simulink model "Ford_T3T6_ArchCnctnDigrm"  (R2016b)
settings: Solver=FixedStepDiscrete  StartTime=0.0  StopTime=10.0  RelTol=1e-3  EnableMultiTasking=on
libraries: canmsglib x15
(part 6 of 15)

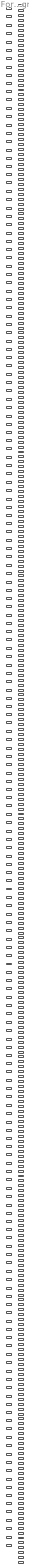
== system Ford_T3T6_ArchCnctnDigrm/Motor Control Manager/AR300FORDA_MotCtrlMgr ==
  AdcDiagcEndPtrOutp : Inport
  AdcDiagcStrtPtrOutp : Inport  Port=2
  BrdgVltg : Inport  Port=3
  CtrlrTFild : Inport  Port=4
  CurrMeasCorrlnSts : Inport  Port=5
  CurrMeasLoaMtgtnEna : Inport  Port=6
  DiagcStsIvtr1Inactv : Inport  Port=7
  DiagcStsIvtr2Inactv : Inport  Port=8
  DualEcuMotCtrlMtgtnEna : Inport  Port=9
  EcuTFild : Inport  Port=10
  HwTq4Raw : Inport  Port=11
  HwTq5Raw : Inport  Port=12
  IvtrFetFltPha : Inport  Port=13
  IvtrFetFltTyp : Inport  Port=14
  IvtrLoaMtgtnEna : Inport  Port=15
  LoopCntr2MilliSec : Inport  Port=16
  MfgEnaSt : Inport  Port=17
  MotAg0ABIFaild : Inport  Port=18
  MotAg0Offs : Inport  Port=19
  MotAg0QepFaild : Inport  Port=20
  MotAg1ABIFaild : Inport  Port=21
  MotAg1Offs : Inport  Port=22
  MotAg1QepFaild : Inport  Port=23
  MotAg2Cos : Inport  Port=24
  MotAg2CosAdcFaild : Inport  Port=25
  MotAg2Sin : Inport  Port=26
  MotAg2SinAdcFaild : Inport  Port=27
  MotAg5CosAdcFaild : Inport  Port=28
  MotAg5CosRtAmpRecpr : Inport  Port=29
  MotAg5CosRtAmpRecpr1 : Inport  Port=30
  MotAg5CosRtOffs : Inport  Port=31
  MotAg5CosRtOffs1 : Inport  Port=32
  MotAg5Polarity : Inport  Port=33
  MotAg5SinAdcFaild : Inport  Port=34
  MotAg5SinRtAmpRecpr : Inport  Port=35
  MotAg5SinRtAmpRecpr1 : Inport  Port=36
  MotAg5SinRtOffs : Inport  Port=37
  MotAg5SinRtOffs1 : Inport  Port=38
  MotAg6CosAdcFaild : Inport  Port=39
  MotAg6CosRtAmpRecpr : Inport  Port=40
  MotAg6CosRtAmpRecpr1 : Inport  Port=41
  MotAg6CosRtOffs : Inport  Port=42
  MotAg6CosRtOffs1 : Inport  Port=43
  MotAg6Polarity : Inport  Port=44
  MotAg6SinAdcFaild : Inport  Port=45
  MotAg6SinRtAmpRecpr : Inport  Port=46
  MotAg6SinRtAmpRecpr1 : Inport  Port=47
  MotAg6SinRtOffs : Inport  Port=48
  MotAg6SinRtOffs1 : Inport  Port=49
  MotAgAMecl : Inport  Port=50
  MotAgAMeclQlfr : Inport  Port=51
  MotAgAMeclRollgCntr : Inport  Port=52
  MotAgBMecl : Inport  Port=53
  MotAgBMeclQlfr : Inport  Port=54
  MotAgBMeclRollgCntr : Inport  Port=55
  MotAgBuf_SigIn : Inport  Port=56
  MotAgCorrd : Inport  Port=57
  MotAgElecDly : Inport  Port=58
  MotAgElecDlyRpl : Inport  Port=59
  MotAgMecl0Polarity : Inport  Port=60
  MotAgMecl1Polarity : Inport  Port=61
  MotAgMeclCorrlnSt : Inport  Port=62
  MotAgMeclCorrlnSts : Inport  Port=63
  MotAgTiBuf_SigIn : Inport  Port=64
  MotAndThermProtnLoaMod : Inport  Port=65
  MotCurrAdcVlyAAdcFaild : Inport  Port=66
  MotCurrAdcVlyBAdcFaild : Inport  Port=67
  MotCurrAdcVlyCAdcFaild : Inport  Port=68
  MotCurrAdcVlyDAdcFaild : Inport  Port=69
  MotCurrAdcVlyEAdcFaild : Inport  Port=70
  MotCurrAdcVlyFAdcFaild : Inport  Port=71
  MotCurrCmd : Inport  Port=72
  MotCurrDaxCmd : Inport  Port=73
  MotCurrDaxMax : Inport  Port=74
  MotCurrEolCalSt : Inport  Port=75
  MotCurrLoaMtgtnEna : Inport  Port=76
  MotCurrQaxCmd : Inport  Port=77
  MotCurrQaxToMotTqGain : Inport  Port=78
  MotDampgDax : Inport  Port=79
  MotDampgQax : Inport  Port=80
  MotElecMeclPolarity : Inport  Port=81
  MotIntglGain : Inport  Port=82
  MotIntglGainDax : Inport  Port=83
  MotIntglGainQax : Inport  Port=84
  MotPropGain : Inport  Port=85
  MotPropGainDax : Inport  Port=86
  MotPropGainQax : Inport  Port=87
  MotREstimd : Inport  Port=88
  MotReacncDax : Inport  Port=89
  MotReacncQax : Inport  Port=90
  MotTqRplCoggOrder1Mgn : Inport  Port=91
  MotTqRplCoggOrder1Pha : Inport  Port=92
  MotTqRplCoggOrder2Mgn : Inport  Port=93
  MotTqRplCoggOrder2Pha : Inport  Port=94
  MotTqRplCoggOrder3Mgn : Inport  Port=95
  MotTqRplCoggOrder3Pha : Inport  Port=96
  MotVelMrf : Inport  Port=97
  MotVltgDaxFf : Inport  Port=98
  MotVltgQaxFf : Inport  Port=99
  PhaDiscnctDiagcActv : Inport  Port=100
  PhaDiscnctDiagcPwmVect : Inport  Port=101
  SampleRdyFlgInp : Inport  Port=102
  StrtUpSt : Inport  Port=103
  SysSt : Inport  Port=104
  VehSpd : Inport  Port=105
  MotCtrlAdc0DynRef : Inport  Port=106
  MotCtrlAdc0SelfDiag0 : Inport  Port=107
  MotCtrlAdc0SelfDiag2 : Inport  Port=108
  MotCtrlAdc0SelfDiag4 : Inport  Port=109
  MotCtrlBattRtnCurrAdcFaild : Inport  Port=110
  MotCtrlBattRtnCurrAmprFastLoop : Inport  Port=111
  MotCtrlBattVltgAdc : Inport  Port=112
  MotCtrlBattVltgAdcFaild : Inport  Port=113
  MotCtrlCmuOffs : Inport  Port=114
  MotCtrlFastLoopCntr : Inport  Port=115
  MotCtrlHwTq0Idx : Inport  Port=116
  MotCtrlHwTq0MissErrCntr : Inport  Port=117
  MotCtrlHwTq0SentComSts : Inport  Port=118
  MotCtrlHwTq0SentData : Inport  Port=119
  MotCtrlHwTq2Idx : Inport  Port=120
  MotCtrlHwTq2MissErrCntr : Inport  Port=121
  MotCtrlHwTq2SentComSts : Inport  Port=122
  MotCtrlHwTq2SentData : Inport  Port=123
  MotCtrlHwTq4Buf : Inport  Port=124
  MotCtrlHwTq4RawAdc : Inport  Port=125
  MotCtrlHwTq4RawAdcFaild : Inport  Port=126
  MotCtrlHwTq4RawFastAdcBuf : Inport  Port=127
  MotCtrlHwTq5Buf : Inport  Port=128
  MotCtrlHwTq5RawAdc : Inport  Port=129
  MotCtrlHwTq5RawAdcFaild : Inport  Port=130
  MotCtrlHwTq5RawFastAdcBuf : Inport  Port=131
  MotCtrlHwTq8Idx : Inport  Port=132
  MotCtrlHwTq8MissErrCntr : Inport  Port=133
  MotCtrlHwTq8SentComSts : Inport  Port=134
  MotCtrlHwTq8SentData : Inport  Port=135
  MotCtrlMotAg0ErrReg : Inport  Port=136
  MotCtrlMotAg0Mecl : Inport  Port=137
  MotCtrlMotAg0MeclRollgCntr : Inport  Port=138
  MotCtrlMotAg0ParFltCnt : Inport  Port=139
  MotCtrlMotAg0RawMecl : Inport  Port=140
  MotCtrlMotAg0SpiMecl : Inport  Port=141
  MotCtrlMotAg0TurnCntrReg : Inport  Port=142
  MotCtrlMotAg0VltgFltCnt : Inport  Port=143
  MotCtrlMotAg0WarnReg : Inport  Port=144
  MotCtrlMotAg1ErrReg : Inport  Port=145
  MotCtrlMotAg1Mecl : Inport  Port=146
  MotCtrlMotAg1MeclRollgCntr : Inport  Port=147
  MotCtrlMotAg1ParFltCnt : Inport  Port=148
  MotCtrlMotAg1RawMecl : Inport  Port=149
  MotCtrlMotAg1SpiMecl : Inport  Port=150
  MotCtrlMotAg1TurnCntrReg : Inport  Port=151
  MotCtrlMotAg1VltgFltCnt : Inport  Port=152
  MotCtrlMotAg1WarnReg : Inport  Port=153
  MotCtrlMotAg3Mecl : Inport  Port=154
  MotCtrlMotAg4Mecl : Inport  Port=155
  MotCtrlMotAg5MeasTi : Inport  Port=156
  MotCtrlMotAg5Mecl : Inport  Port=157
  MotCtrlMotAg5RawMecl : Inport  Port=158
  MotCtrlMotAg6MeasTi : Inport  Port=159
  MotCtrlMotAg6Mecl : Inport  Port=160
  MotCtrlMotAg6RawMecl : Inport  Port=161
  MotCtrlMotAgBufIdx : Inport  Port=162
  MotCtrlMotAgBuf_SigOut : Inport  Port=163
  MotCtrlMotAgCumvAlgndMrfRev : Inport  Port=164
  MotCtrlMotAgCumvInid : Inport  Port=165
  MotCtrlMotAgTiBuf_SigOut : Inport  Port=166
  MotCtrlMotCurrAdcPeakA : Inport  Port=167
  MotCtrlMotCurrAdcPeakB : Inport  Port=168
  MotCtrlMotCurrAdcPeakC : Inport  Port=169
  MotCtrlMotCurrAdcPeakD : Inport  Port=170
  MotCtrlMotCurrAdcPeakE : Inport  Port=171
  MotCtrlMotCurrAdcPeakF : Inport  Port=172
  MotCtrlMotCurrQaxCmdFinal : Inport  Port=173
  MotCtrlMotCurrSnsrOffs1 : Inport  Port=174
  MotCtrlMotCurrSnsrOffs2 : Inport  Port=175
  MotCtrlMotVltg : Inport  Port=176
  MotCtrlMotVltgDaxFild : Inport  Port=177
  MotCtrlMotVltgQaxFild : Inport  Port=178
  MotCtrlNtc5DErrCnt : Inport  Port=179
  MotCtrlNtc6DErrCnt : Inport  Port=180
  MotCtrlRegOutpCSIH1RRA : Inport  Port=181
  MotCtrlSampleRdyFlgOutp : Inport  Port=182
  MotCtrlSlowLoopCntr : Inport  Port=183
  MotCtrlTSG31CMP0E : Inport  Port=184
  MotCtrlTSG31CMP12E : Inport  Port=185
  MotCtrlTSG31CMPUE : Inport  Port=186
  Adc0DynRef : Outport
  Adc0RawRes : Outport  Port=2
  Adc0ScanGroup2Ref0 : Outport  Port=3
  Adc0ScanGroup2Ref1 : Outport  Port=4
  Adc0ScanGroup3Ref0 : Outport  Port=5
  Adc0ScanGroup3Ref1 : Outport  Port=6
  Adc0SelfDiag0 : Outport  Port=7
  Adc0SelfDiag2 : Outport  Port=8
  Adc0SelfDiag4 : Outport  Port=9
  Adc1RawRes : Outport  Port=10
  BattRtnCurrAdc : Outport  Port=11
  BattRtnCurrAdcFaild : Outport  Port=12
  BattRtnCurrAmprFastLoop : Outport  Port=13
  BattVltgAdc : Outport  Port=14
  BattVltgAdcFaild : Outport  Port=15
  CmuOffs : Outport  Port=16
  CurrMeasMotAgCorrd : Outport  Port=17
  CurrMeasWrmIninTestCmpl : Outport  Port=18
  EcuId : Outport  Port=19
  FastLoopCntr : Outport  Port=20
  HwTq0Idx : Outport  Port=21
  HwTq0MissErrCntr : Outport  Port=22
  HwTq0SentComSts : Outport  Port=23
  HwTq0SentData : Outport  Port=24
  HwTq2Idx : Outport  Port=25
  HwTq2MissErrCntr : Outport  Port=26
  HwTq2SentComSts : Outport  Port=27
  HwTq2SentData : Outport  Port=28
  HwTq4Buf : Outport  Port=29
  HwTq4RawAdc : Outport  Port=30
  HwTq4RawAdcFaild : Outport  Port=31
  HwTq4RawFastAdc : Outport  Port=32
  HwTq4RawFastAdcBuf : Outport  Port=33
  HwTq5Buf : Outport  Port=34
  HwTq5RawAdc : Outport  Port=35
  HwTq5RawAdcFaild : Outport  Port=36
  HwTq5RawFastAdc : Outport  Port=37
  HwTq5RawFastAdcBuf : Outport  Port=38
  HwTq8Idx : Outport  Port=39
  HwTq8MissErrCntr : Outport  Port=40
  HwTq8SentComSts : Outport  Port=41
  HwTq8SentData : Outport  Port=42
  MotAg0ErrReg : Outport  Port=43
  MotAg0Mecl : Outport  Port=44
  MotAg0MeclRollgCntr : Outport  Port=45
  MotAg0ParFltCnt : Outport  Port=46
  MotAg0RawMecl : Outport  Port=47
  MotAg0RawRes : Outport  Port=48
  MotAg0SpiMecl : Outport  Port=49
  MotAg0TurnCntrReg : Outport  Port=50
  MotAg0VltgFltCnt : Outport  Port=51
  MotAg0WarnReg : Outport  Port=52
  MotAg1ErrReg : Outport  Port=53
  MotAg1Mecl : Outport  Port=54
  MotAg1MeclRollgCntr : Outport  Port=55
  MotAg1ParFltCnt : Outport  Port=56
  MotAg1RawMecl : Outport  Port=57
  MotAg1RawRes : Outport  Port=58
  MotAg1SpiMecl : Outport  Port=59
  MotAg1TurnCntrReg : Outport  Port=60
  MotAg1VltgFltCnt : Outport  Port=61
  MotAg1WarnReg : Outport  Port=62
  MotAg3Mecl : Outport  Port=63
  MotAg4Mecl : Outport  Port=64
  MotAg5Cos : Outport  Port=65
  MotAg5MeasTi : Outport  Port=66
  MotAg5Mecl : Outport  Port=67
  MotAg5RawMecl : Outport  Port=68
  MotAg5Sin : Outport  Port=69
  MotAg6Cos : Outport  Port=70
  MotAg6MeasTi : Outport  Port=71
  MotAg6Mecl : Outport  Port=72
  MotAg6RawMecl : Outport  Port=73
  MotAg6Sin : Outport  Port=74
  MotAgBuf : Outport  Port=75
  MotAgBufIdx : Outport  Port=76
  MotAgBuf_SigOut : Outport  Port=77
  MotAgCumvAlgndMrfRev : Outport  Port=78
  MotAgCumvInid : Outport  Port=79
  MotAgElec : Outport  Port=80
  MotAgMeasTi : Outport  Port=81
  MotAgMecl : Outport  Port=82
  MotAgTiBuf : Outport  Port=83
  MotAgTiBuf_SigOut : Outport  Port=84
  MotBackEmfVltg : Outport  Port=85
  MotCurr : Outport  Port=86
  MotCurrAdcPeakA : Outport  Port=87
  MotCurrAdcPeakB : Outport  Port=88
  MotCurrAdcPeakC : Outport  Port=89
  MotCurrAdcPeakD : Outport  Port=90
  MotCurrAdcPeakE : Outport  Port=91
  MotCurrAdcPeakF : Outport  Port=92
  MotCurrAdcVlyA : Outport  Port=93
  MotCurrAdcVlyB : Outport  Port=94
  MotCurrAdcVlyC : Outport  Port=95
  MotCurrAdcVlyD : Outport  Port=96
  MotCurrAdcVlyE : Outport  Port=97
  MotCurrAdcVlyF : Outport  Port=98
  MotCurrCorrdA : Outport  Port=99
  MotCurrCorrdB : Outport  Port=100
  MotCurrCorrdC : Outport  Port=101
  MotCurrCorrdD : Outport  Port=102
  MotCurrCorrdE : Outport  Port=103
  MotCurrCorrdF : Outport  Port=104
  MotCurrDax : Outport  Port=105
  MotCurrQax : Outport  Port=106
  MotCurrQaxCmdFinal : Outport  Port=107
  MotCurrQaxCoggCmd : Outport  Port=108
  MotCurrQaxRplCmd : Outport  Port=109
  MotCurrQlfr1 : Outport  Port=110
  MotCurrQlfr2 : Outport  Port=111
  MotCurrRollgCntr1 : Outport  Port=112
  MotCurrRollgCntr2 : Outport  Port=113
  MotCurrSnsrOffs1 : Outport  Port=114
  MotCurrSnsrOffs2 : Outport  Port=115
  MotInduDaxEstimdIvs : Outport  Port=116
  MotInduQaxEstimdIvs : Outport  Port=117
  MotModlnIdx : Outport  Port=118
  MotPhaAdv : Outport  Port=119
  MotVltg : Outport  Port=120
  MotVltgCmdPolarity : Outport  Port=121
  MotVltgDax : Outport  Port=122
  MotVltgDaxFild : Outport  Port=123
  MotVltgQax : Outport  Port=124
  MotVltgQaxFild : Outport  Port=125
  Ntc5DErrCnt : Outport  Port=126
  Ntc6DErrCnt : Outport  Port=127
  PhaOnTiA : Outport  Port=128
  PhaOnTiB : Outport  Port=129
  PhaOnTiC : Outport  Port=130
  PhaOnTiSumA : Outport  Port=131
  PhaOnTiSumB : Outport  Port=132
  PhaOnTiSumC : Outport  Port=133
  PwmPerd : Outport  Port=134
  RegOutpCSIH1RRA : Outport  Port=135
  SampleRdyFlgOutp : Outport  Port=136
  SlowLoopCntr : Outport  Port=137
  SwCalEna : Outport  Port=138
  SwCalModlnIdx : Outport  Port=139
  SwCalPosnIdx : Outport  Port=140
  TSG31CMP0E : Outport  Port=141
  TSG31CMP12E : Outport  Port=142
  TSG31CMPUE : Outport  Port=143
  TSG31CMPVE : Outport  Port=144
  TSG31CMPWE : Outport  Port=145
  TSG31DCMP0E : Outport  Port=146
  MotCtrlAdc0RawRes : Outport  Port=147
  MotCtrlAdc0ScanGroup2Ref0 : Outport  Port=148
  MotCtrlAdc0ScanGroup2Ref1 : Outport  Port=149
  MotCtrlAdc0ScanGroup3Ref0 : Outport  Port=150
  MotCtrlAdc0ScanGroup3Ref1 : Outport  Port=151
  MotCtrlAdc1RawRes : Outport  Port=152
  MotCtrlAdcDiagcEndPtrOutp : Outport  Port=153
  MotCtrlAdcDiagcStrtPtrOutp : Outport  Port=154
  MotCtrlBattRtnCurrAdc : Outport  Port=155
  MotCtrlBrdgVltg : Outport  Port=156
  MotCtrlCtrlrTFild : Outport  Port=157
  MotCtrlCurrMeasCorrlnSts : Outport  Port=158
  MotCtrlCurrMeasLoaMtgtnEna : Outport  Port=159
  MotCtrlCurrMeasMotAgCorrd : Outport  Port=160
  MotCtrlCurrMeasWrmIninTestCmpl : Outport  Port=161
  MotCtrlDiagcStsIvtr1Inactv : Outport  Port=162
  MotCtrlDiagcStsIvtr2Inactv : Outport  Port=163
  MotCtrlDualEcuMotCtrlMtgtnEna : Outport  Port=164
  MotCtrlEcuTFild : Outport  Port=165
  MotCtrlHwTq4Raw : Outport  Port=166
  MotCtrlHwTq4RawFastAdc : Outport  Port=167
  MotCtrlHwTq5Raw : Outport  Port=168
  MotCtrlHwTq5RawFastAdc : Outport  Port=169
  MotCtrlIvtrFetFltPha : Outport  Port=170
  MotCtrlIvtrFetFltTyp : Outport  Port=171
  MotCtrlIvtrLoaMtgtnEna : Outport  Port=172
  MotCtrlLoopCntr2MilliSec : Outport  Port=173
  MotCtrlMfgEnaSt : Outport  Port=174
  MotCtrlMotAg0ABIFaild : Outport  Port=175
  MotCtrlMotAg0Offs : Outport  Port=176
  MotCtrlMotAg0QepFaild : Outport  Port=177
  MotCtrlMotAg0RawRes : Outport  Port=178
  MotCtrlMotAg1ABIFaild : Outport  Port=179
  MotCtrlMotAg1Offs : Outport  Port=180
  MotCtrlMotAg1QepFaild : Outport  Port=181
  MotCtrlMotAg1RawRes : Outport  Port=182
  MotCtrlMotAg2Cos : Outport  Port=183
  MotCtrlMotAg2CosAdcFaild : Outport  Port=184
  MotCtrlMotAg2Sin : Outport  Port=185
  MotCtrlMotAg2SinAdcFaild : Outport  Port=186
  MotCtrlMotAg5Cos : Outport  Port=187
  MotCtrlMotAg5CosAdcFaild : Outport  Port=188
  MotCtrlMotAg5CosRtAmpRecpr : Outport  Port=189
  MotCtrlMotAg5CosRtAmpRecpr1 : Outport  Port=190
  MotCtrlMotAg5CosRtOffs : Outport  Port=191
  MotCtrlMotAg5CosRtOffs1 : Outport  Port=192
  MotCtrlMotAg5Polarity : Outport  Port=193
  MotCtrlMotAg5Sin : Outport  Port=194
  MotCtrlMotAg5SinAdcFaild : Outport  Port=195
  MotCtrlMotAg5SinRtAmpRecpr : Outport  Port=196
  MotCtrlMotAg5SinRtAmpRecpr1 : Outport  Port=197
  MotCtrlMotAg5SinRtOffs : Outport  Port=198
  MotCtrlMotAg5SinRtOffs1 : Outport  Port=199
  MotCtrlMotAg6Cos : Outport  Port=200
  MotCtrlMotAg6CosAdcFaild : Outport  Port=201
  MotCtrlMotAg6CosRtAmpRecpr : Outport  Port=202
  MotCtrlMotAg6CosRtAmpRecpr1 : Outport  Port=203
  MotCtrlMotAg6CosRtOffs : Outport  Port=204
  MotCtrlMotAg6CosRtOffs1 : Outport  Port=205
  MotCtrlMotAg6Polarity : Outport  Port=206
  MotCtrlMotAg6Sin : Outport  Port=207
  MotCtrlMotAg6SinAdcFaild : Outport  Port=208
  MotCtrlMotAg6SinRtAmpRecpr : Outport  Port=209
  MotCtrlMotAg6SinRtAmpRecpr1 : Outport  Port=210
  MotCtrlMotAg6SinRtOffs : Outport  Port=211
  MotCtrlMotAg6SinRtOffs1 : Outport  Port=212
  MotCtrlMotAgAMecl : Outport  Port=213
  MotCtrlMotAgAMeclQlfr : Outport  Port=214
  MotCtrlMotAgAMeclRollgCntr : Outport  Port=215
  MotCtrlMotAgBMecl : Outport  Port=216
  MotCtrlMotAgBMeclQlfr : Outport  Port=217
  MotCtrlMotAgBMeclRollgCntr : Outport  Port=218
  MotCtrlMotAgBuf : Outport  Port=219
  MotCtrlMotAgBuf_SigIn : Outport  Port=220
  MotCtrlMotAgCorrd : Outport  Port=221
  MotCtrlMotAgElec : Outport  Port=222
  MotCtrlMotAgElecDly : Outport  Port=223
  MotCtrlMotAgElecDlyRpl : Outport  Port=224
  MotCtrlMotAgMeasTi : Outport  Port=225
  MotCtrlMotAgMecl : Outport  Port=226
  MotCtrlMotAgMecl0Polarity : Outport  Port=227
  MotCtrlMotAgMecl1Polarity : Outport  Port=228
  MotCtrlMotAgMeclCorrlnSt : Outport  Port=229
  MotCtrlMotAgMeclCorrlnSts : Outport  Port=230
  MotCtrlMotAgTiBuf : Outport  Port=231
  MotCtrlMotAgTiBuf_SigIn : Outport  Port=232
  MotCtrlMotAndThermProtnLoaMod : Outport  Port=233
  MotCtrlMotBackEmfVltg : Outport  Port=234
  MotCtrlMotCurr : Outport  Port=235
  MotCtrlMotCurrAdcVlyA : Outport  Port=236
  MotCtrlMotCurrAdcVlyAAdcFaild : Outport  Port=237
  MotCtrlMotCurrAdcVlyB : Outport  Port=238
  MotCtrlMotCurrAdcVlyBAdcFaild : Outport  Port=239
  MotCtrlMotCurrAdcVlyC : Outport  Port=240
  MotCtrlMotCurrAdcVlyCAdcFaild : Outport  Port=241
  MotCtrlMotCurrAdcVlyD : Outport  Port=242
  MotCtrlMotCurrAdcVlyDAdcFaild : Outport  Port=243
  MotCtrlMotCurrAdcVlyE : Outport  Port=244
  MotCtrlMotCurrAdcVlyEAdcFaild : Outport  Port=245
  MotCtrlMotCurrAdcVlyF : Outport  Port=246
  MotCtrlMotCurrAdcVlyFAdcFaild : Outport  Port=247
  MotCtrlMotCurrCmd : Outport  Port=248
  MotCtrlMotCurrCorrdA : Outport  Port=249
  MotCtrlMotCurrCorrdB : Outport  Port=250
  MotCtrlMotCurrCorrdC : Outport  Port=251
  MotCtrlMotCurrCorrdD : Outport  Port=252
  MotCtrlMotCurrCorrdE : Outport  Port=253
  MotCtrlMotCurrCorrdF : Outport  Port=254
  MotCtrlMotCurrDax : Outport  Port=255
  MotCtrlMotCurrDaxCmd : Outport  Port=256
  MotCtrlMotCurrDaxMax : Outport  Port=257
  MotCtrlMotCurrEolCalSt : Outport  Port=258
  MotCtrlMotCurrLoaMtgtnEna : Outport  Port=259
  MotCtrlMotCurrQax : Outport  Port=260
  MotCtrlMotCurrQaxCmd : Outport  Port=261
  MotCtrlMotCurrQaxCoggCmd : Outport  Port=262
  MotCtrlMotCurrQaxRplCmd : Outport  Port=263
  MotCtrlMotCurrQaxToMotTqGain : Outport  Port=264
  MotCtrlMotCurrQlfr1 : Outport  Port=265
  MotCtrlMotCurrQlfr2 : Outport  Port=266
  MotCtrlMotCurrRollgCntr1 : Outport  Port=267
  MotCtrlMotCurrRollgCntr2 : Outport  Port=268
  MotCtrlMotDampgDax : Outport  Port=269
  MotCtrlMotDampgQax : Outport  Port=270
  MotCtrlMotElecMeclPolarity : Outport  Port=271
  MotCtrlMotInduDaxEstimdIvs : Outport  Port=272
  MotCtrlMotInduQaxEstimdIvs : Outport  Port=273
  MotCtrlMotIntglGain : Outport  Port=274
  MotCtrlMotIntglGainDax : Outport  Port=275
  MotCtrlMotIntglGainQax : Outport  Port=276
  MotCtrlMotModlnIdx : Outport  Port=277
  MotCtrlMotPhaAdv : Outport  Port=278
  MotCtrlMotPropGain : Outport  Port=279
  MotCtrlMotPropGainDax : Outport  Port=280
  MotCtrlMotPropGainQax : Outport  Port=281
  MotCtrlMotREstimd : Outport  Port=282
  MotCtrlMotReacncDax : Outport  Port=283
  MotCtrlMotReacncQax : Outport  Port=284
  MotCtrlMotTqRplCoggOrder1Mgn : Outport  Port=285
  MotCtrlMotTqRplCoggOrder1Pha : Outport  Port=286
  MotCtrlMotTqRplCoggOrder2Mgn : Outport  Port=287
  MotCtrlMotTqRplCoggOrder2Pha : Outport  Port=288
  MotCtrlMotTqRplCoggOrder3Mgn : Outport  Port=289
  MotCtrlMotTqRplCoggOrder3Pha : Outport  Port=290
  MotCtrlMotVelMrf : Outport  Port=291
  MotCtrlMotVltgCmdPolarity : Outport  Port=292
  MotCtrlMotVltgDax : Outport  Port=293
  MotCtrlMotVltgDaxFf : Outport  Port=294
  MotCtrlMotVltgQax : Outport  Port=295
  MotCtrlMotVltgQaxFf : Outport  Port=296
  MotCtrlPhaDiscnctDiagcActv : Outport  Port=297
  MotCtrlPhaDiscnctDiagcPwmVect : Outport  Port=298
  MotCtrlPhaOnTiA : Outport  Port=299
  MotCtrlPhaOnTiB : Outport  Port=300
  MotCtrlPhaOnTiC : Outport  Port=301
  MotCtrlPhaOnTiSumA : Outport  Port=302
  MotCtrlPhaOnTiSumB : Outport  Port=303
  MotCtrlPhaOnTiSumC : Outport  Port=304
  MotCtrlPwmPerd : Outport  Port=305
  MotCtrlSampleRdyFlgInp : Outport  Port=306
  MotCtrlStrtUpSt : Outport  Port=307
  MotCtrlSwCalEna : Outport  Port=308
  MotCtrlSwCalModlnIdx : Outport  Port=309
  MotCtrlSwCalPosnIdx : Outport  Port=310
  MotCtrlSysSt : Outport  Port=311
  MotCtrlTSG31CMPVE : Outport  Port=312
  MotCtrlTSG31CMPWE : Outport  Port=313
  MotCtrlTSG31DCMP0E : Outport  Port=314
  MotCtrlVehSpd : Outport  Port=315

== system Ford_T3T6_ArchCnctnDigrm/States and Modes/ES002A_McuDiagc ==
  FastLoopCntr : Inport
  SlowLoopCntr : Inport  Port=2
  SysSt : Inport  Port=3
  MotCtrlLoopCntr2MilliSec : Inport  Port=4
  ReadErrInjReg : Inport  Port=5
  SetNtcSts : Inport  Port=6
  StrtErrInjCntr : Inport  Port=7
  LoopCntr2MilliSec : Outport
  MotCtrlFastLoopCntr : Outport  Port=2
  MotCtrlSlowLoopCntr : Outport  Port=3

== system Ford_T3T6_ArchCnctnDigrm/States and Modes/ES100A_SysStMod ==
  PwrSplyEnaReq : Inport
  SysStFltOutpReqDi : Inport  Port=2
  SysStImdtTranReqOff : Inport  Port=3
  SysStReqDi : Inport  Port=4
  SysStReqEna : Inport  Port=5
  SysStWrmIninCmpl : Inport  Port=6
  StrtUpSt : Inport  Port=7
  SysSt : Outport

== system Ford_T3T6_ArchCnctnDigrm/States and Modes/SF048A_TqLoa ==
  MotAgLoaMtgtnEna : Inport
  MotVelCrf : Inport  Port=2
  PinionAg : Inport  Port=3
  PinionAgConf : Inport  Port=4
  VehLatA : Inport  Port=5
  VehLatAVld : Inport  Port=6
  VehSpd : Inport  Port=7
  VehSpdVld : Inport  Port=8
  TqLoaAvl : Outport
  TqLoaCmd : Outport  Port=2

== system Ford_T3T6_ArchCnctnDigrm/States and Modes/SF049B_LoaMgr ==
  CurrMeasIdptSig : Inport
  DiagcStsIvtr1Inactv : Inport  Port=2
  DiagcStsIvtr2Inactv : Inport  Port=3
  HwTqIdptSig : Inport  Port=4
  IvtrFetFltTyp : Inport  Port=5
  LoaScaDi : Inport  Port=6
  MotAgMeclIdptSig : Inport  Port=7
  MotAgSnsrlsAvl : Inport  Port=8
  TqLoaAvl : Inport  Port=9
  VehSteerMod : Inport  Port=10
  SetNtcSts : Inport  Port=11
  HwTqLoaMtgtnEna : Outport
  LoaRateLim : Outport  Port=2
  LoaSca : Outport  Port=3
  LoaSt : Outport  Port=4
  MotAgLoaMtgtnEna : Outport  Port=5
  MotAndThermProtnLoaMod : Outport  Port=6

== system Ford_T3T6_ArchCnctnDigrm/States and Modes/SystemStartUpState ==
  note: es003c update need from ES
  note: More like microdiagc
  note: ASIL D
  note: ASIL D
  note: ASIL D Safety Mech
  note: ASIL B
  note: ASIL B
  note: ASIL D Safety Mech
  SysSt : Inport
  ES003C_PwrDiscnct : Subsystem  Tag=2.0.0  Description=Power Disconnect with Bridge,Single Inverter and No Precharge
      settings: AttributesFormatString=Version: %<Tag>
  ES004A_PwrUpSeq : Subsystem  Tag=2.0.0  Description=Determine if the System State WarmInit Milestones have been completed or not.
      settings: AttributesFormatString=Version: %<Tag>
  ES005C_TmplMonr : Subsystem  Tag=1.1.0  Description=Temporal Monitor Function
      settings: AttributesFormatString=Version: %<Tag>
  ES008A_PwrSply : Subsystem  Tag=1.7.0  Description=Power Supply Diagnostics Function
      settings: AttributesFormatString=Version: %<Tag>
  ES108A_ShtdwnMech : Subsystem  Tag=1.0.2  Description=Shutdown Mechanism Single Inverter
      settings: AttributesFormatString=Version: %<Tag>
  ES311A_GateDrv0Ctrl : Subsystem  Tag=3.2.0  Description=Function responsible for configuration, deactivation and determination of fault status of the Gate Drive 0
      settings: AttributesFormatString=Version: %<Tag>
  SysStWrmIninCmpl : Outport
  StrtUpSt : Outport  Port=2
  tag scope: DiagcStsIvtr1Inactv=global, Ivtr1PwrDiscnctFltSts=global, IvtrFetFltPha=global, IvtrFetFltTyp=global, MotDrvErrA=global, MotDrvErrB=global, MotDrvErrC=global, PwrDiscnctATestCmpl=global, PwrDiscnctBTestCmpl=global, PwrTurnOffCtrl=global, StrtUpSt=global, SysStWrmIninCmpl=global
  wires:
  ES004A_PwrUpSeq/2(SysStWrmIninCmpl) -> SysStWrmIninCmpl/1, [SysStWrmIninCmpl]
  [SysSt] -> ES008A_PwrSply/1(SysSt)
  [Spi_GetSequenceResult] -> ES008A_PwrSply/2(Spi_GetSequenceResult)
  [Call_Spi_AsyncTransmit] -> ES008A_PwrSply/3(Call_Spi_AsyncTransmit)
  [SetNtcSts8] -> ES008A_PwrSply/4(SetNtcSts)
  [Spi_ReadIB] -> ES008A_PwrSply/5(Spi_ReadIB)
  [Spi_WriteIB] -> ES008A_PwrSply/6(Spi_WriteIB)
  [CodFlsCrcChkCmpl] -> ES004A_PwrUpSeq/1(CodFlsCrcChkCmpl)
  [CurrMeasWrmIninTestCmpl] -> ES004A_PwrUpSeq/2(CurrMeasWrmIninTestCmpl)
  ES311A_GateDrv0Ctrl/7(MotDrvr0IninTestCmpl) -> ES004A_PwrUpSeq/3(MotDrvr0IninTestCmpl)
  [MotDrvr1IninTestCmpl] -> ES004A_PwrUpSeq/4(MotDrvr1IninTestCmpl)
  [PhaDiscnctWrmIninTestCmpl] -> ES004A_PwrUpSeq/5(PhaDiscnctWrmIninTestCmpl)
  ES003C_PwrDiscnct/2(PwrDiscnctATestCmpl) -> ES004A_PwrUpSeq/6(PwrDiscnctATestCmpl), [PwrDiscnctATestCmpl]
  ES003C_PwrDiscnct/3(PwrDiscnctBTestCmpl) -> ES004A_PwrUpSeq/7(PwrDiscnctBTestCmpl), [PwrDiscnctBTestCmpl]
  ES005C_TmplMonr/1(TmplMonrIninTestCmpl) -> ES004A_PwrUpSeq/9(TmplMonIninTestCmpl)
  [IoHwAb_SetGpioPwrTurnOffCtrl] -> ES004A_PwrUpSeq/10(IoHwAb_SetGpioPwrTurnOffCtrl)
  ES004A_PwrUpSeq/3(PwrTurnOffCtrl) -> [PwrTurnOffCtrl]
  [BattVltg] -> ES003C_PwrDiscnct/1(BattVltg)
  [BattVltgAdcFaild] -> ES003C_PwrDiscnct/2(BattVltgAdcFaild)
  [BattVltgSwd1] -> ES003C_PwrDiscnct/3(BattVltgSwd1)
  [ChrgPmpDiag] -> ES003C_PwrDiscnct/4(ChrgPmpDiag)
  [ChrgPmpDiagAdcFaild] -> ES003C_PwrDiscnct/5(ChrgPmpDiagAdcFaild)
  [MotVelMrf] -> ES003C_PwrDiscnct/6(MotVelMrf)
  [PwrDiscnctSwtDiag] -> ES003C_PwrDiscnct/7(PwrDiscnctSwtDiag)
  [SysSt] -> ES003C_PwrDiscnct/9(SysSt)
  [CnvSnpshtData_f32] -> ES003C_PwrDiscnct/10(CnvSnpshtData_f32)
  [GetNtcQlfrSts9] -> ES003C_PwrDiscnct/11(GetNtcQlfrSts)
  [SetNtcStsAndSnpshtData9] -> ES003C_PwrDiscnct/12(SetNtcStsAndSnpshtData)
  ES003C_PwrDiscnct/1(Ivtr1PwrDiscnctFltSts) -> [Ivtr1PwrDiscnctFltSts]
  [DiagcStsIvtr1Inactv] -> ES108A_ShtdwnMech/1(DiagcStsIvtr1Inactv)
  [StrtUpSt] -> ES108A_ShtdwnMech/2(StrtUpSt)
  [IoHwAb_SetGpioSysFlt2A] -> ES108A_ShtdwnMech/3(IoHwAb_SetGpioSysFlt2A)
  [Ivtr1PwrDiscnctFltSts] -> ES311A_GateDrv0Ctrl/1(Ivtr1PwrDiscnctFltSts)
  [PhaOnTiMeasdA] -> ES311A_GateDrv0Ctrl/2(PhaOnTiMeasdA)
  [PhaOnTiMeasdB] -> ES311A_GateDrv0Ctrl/3(PhaOnTiMeasdB)
  [PhaOnTiMeasdC] -> ES311A_GateDrv0Ctrl/4(PhaOnTiMeasdC)
  [PhaOnTiSumA] -> ES311A_GateDrv0Ctrl/5(PhaOnTiSumA)
  [PhaOnTiSumB] -> ES311A_GateDrv0Ctrl/6(PhaOnTiSumB)
  [PhaOnTiSumC] -> ES311A_GateDrv0Ctrl/7(PhaOnTiSumC)
  [Call_Spi_AsyncTransmit] -> ES311A_GateDrv0Ctrl/10(Call_Spi_AsyncTransmit)
  [GetNtcQlfrSts] -> ES311A_GateDrv0Ctrl/11(GetNtcQlfrSts)
  [IoHwAb_GetGpioMotDrvr0Diag] -> ES311A_GateDrv0Ctrl/12(IoHwAb_GetGpioMotDrvr0Diag)
  [IoHwAb_SetGpioGateDrv0Rst] -> ES311A_GateDrv0Ctrl/13(IoHwAb_SetGpioGateDrv0Rst)
  [IoHwAb_SetGpioSysFlt2A] -> ES311A_GateDrv0Ctrl/14(IoHwAb_SetGpioSysFlt2A)
  [SetNtcSts] -> ES311A_GateDrv0Ctrl/15(SetNtcSts)
  [SetNtcStsAndSnpshtData] -> ES311A_GateDrv0Ctrl/16(SetNtcStsAndSnpshtData)
  [Spi_GetSequenceResult] -> ES311A_GateDrv0Ctrl/17(Spi_GetSequenceResult)
  [Spi_ReadIB] -> ES311A_GateDrv0Ctrl/18(Spi_ReadIB)
  [Spi_WriteIB] -> ES311A_GateDrv0Ctrl/19(Spi_WriteIB)
  ES311A_GateDrv0Ctrl/1(DiagcStsIvtr1Inactv) -> [DiagcStsIvtr1Inactv]
  ES311A_GateDrv0Ctrl/2(IvtrFetFltPha) -> [IvtrFetFltPha]
  ES311A_GateDrv0Ctrl/3(IvtrFetFltTyp) -> [IvtrFetFltTyp]
  ES311A_GateDrv0Ctrl/4(MotDrvErrA) -> [MotDrvErrA]
  ES311A_GateDrv0Ctrl/5(MotDrvErrB) -> [MotDrvErrB]
  ES311A_GateDrv0Ctrl/6(MotDrvErrC) -> [MotDrvErrC]
  ES004A_PwrUpSeq/1(StrtUpSt) -> ES003C_PwrDiscnct/8(StrtUpSt), ES005C_TmplMonr/1(StrtUpSt), ES311A_GateDrv0Ctrl/8(StrtUpSt), StrtUpSt/1, [StrtUpSt]
  SysSt/1 -> ES005C_TmplMonr/2(SysSt), ES311A_GateDrv0Ctrl/9(SysSt), ES004A_PwrUpSeq/8(SysSt)
  [Spi_GetSequenceResult] -> ES005C_TmplMonr/3(Spi_GetSequenceResult)
  [Call_Spi_AsyncTransmit] -> ES005C_TmplMonr/4(Call_Spi_AsyncTransmit)
  [CtrlErrOut] -> ES005C_TmplMonr/5(CtrlErrOut)
  [GetRefTmr1MicroSec32bit] -> ES005C_TmplMonr/6(GetRefTmr1MicroSec32bit)
  [GetTiSpan1MicroSec32bit] -> ES005C_TmplMonr/7(GetTiSpan1MicroSec32bit)
  [IoHwAb_GetGpioPwrOutpEnaFb] -> ES005C_TmplMonr/8(IoHwAb_GetGpioPwrOutpEnaFb)
  [IoHwAb_SetGpioTmplMonrWdg] -> ES005C_TmplMonr/9(IoHwAb_SetGpioTmplMonrWdg)
  [SetNtcSts] -> ES005C_TmplMonr/10(SetNtcSts)
  [Spi_ReadIB] -> ES005C_TmplMonr/11(Spi_ReadIB)
  [Spi_WriteIB] -> ES005C_TmplMonr/12(Spi_WriteIB)

== system Ford_T3T6_ArchCnctnDigrm/Support Functions/AR100A_NxtrMath ==
  ReadErrInjReg : Inport
  SetNtcSts : Inport  Port=2
  InjSwFpuErr : Outport
  gh_set_errno : Outport  Port=2

== system Ford_T3T6_ArchCnctnDigrm/Support Functions/AR200A_NxtrSuprt ==

== system Ford_T3T6_ArchCnctnDigrm/Support Functions/AR999A_ArchGlbPrm ==

== system Ford_T3T6_ArchCnctnDigrm/Support Functions/ES101AProxy10_DiagcMgrProxy10 ==
  ClrDiagcFlgProxy : Inport
  DiagcMgrIninCore : Inport  Port=2
  GetNtcActvCore : Inport  Port=3
  GetNtcQlfrStsCore : Inport  Port=4
  GetNtcStsCore : Inport  Port=5
  SetNtcStsCore : Inport  Port=6
  GetDiagcDataAppl10 : Outport
  GetNtcActv10 : Outport  Port=2
  GetNtcDebCntrAppl10 : Outport  Port=3
  GetNtcInfoAppl10 : Outport  Port=4
  GetNtcQlfrSts10 : Outport  Port=5
  GetNtcSts10 : Outport  Port=6
  SetNtcSts10 : Outport  Port=7
  SetNtcStsAndSnpshtData10 : Outport  Port=8

== system Ford_T3T6_ArchCnctnDigrm/Support Functions/ES101AProxy6_DiagcMgrProxy6 ==
  ClrDiagcFlgProxy : Inport
  DiagcMgrIninCore : Inport  Port=2
  GetNtcActvCore : Inport  Port=3
  GetNtcQlfrStsCore : Inport  Port=4
  GetNtcStsCore : Inport  Port=5
  SetNtcStsCore : Inport  Port=6
  GetDiagcDataAppl6 : Outport
  GetNtcActv6 : Outport  Port=2
  GetNtcDebCntrAppl6 : Outport  Port=3
  GetNtcInfoAppl6 : Outport  Port=4
  GetNtcQlfrSts6 : Outport  Port=5
  GetNtcSts6 : Outport  Port=6
  SetNtcSts6 : Outport  Port=7
  SetNtcStsAndSnpshtData6 : Outport  Port=8

== system Ford_T3T6_ArchCnctnDigrm/Support Functions/ES101AProxy7_DiagcMgrProxy7 ==
  ClrDiagcFlgProxy : Inport
  DiagcMgrIninCore : Inport  Port=2
  GetNtcActvCore : Inport  Port=3
  GetNtcQlfrStsCore : Inport  Port=4
  GetNtcStsCore : Inport  Port=5
  SetNtcStsCore : Inport  Port=6
  GetDiagcDataAppl7 : Outport
  GetNtcActv7 : Outport  Port=2
  GetNtcDebCntrAppl7 : Outport  Port=3
  GetNtcInfoAppl7 : Outport  Port=4
  GetNtcQlfrSts7 : Outport  Port=5
  GetNtcSts7 : Outport  Port=6
  SetNtcSts7 : Outport  Port=7
  SetNtcStsAndSnpshtData7 : Outport  Port=8

== system Ford_T3T6_ArchCnctnDigrm/Support Functions/ES101AProxy8_DiagcMgrProxy8 ==
  ClrDiagcFlgProxy : Inport
  DiagcMgrIninCore : Inport  Port=2
  GetNtcActvCore : Inport  Port=3
  GetNtcQlfrStsCore : Inport  Port=4
  GetNtcStsCore : Inport  Port=5
  SetNtcStsCore : Inport  Port=6
  GetDiagcDataAppl8 : Outport
  GetNtcActv8 : Outport  Port=2
  GetNtcDebCntrAppl8 : Outport  Port=3
  GetNtcInfoAppl8 : Outport  Port=4
  GetNtcQlfrSts8 : Outport  Port=5
  GetNtcSts8 : Outport  Port=6
  SetNtcSts8 : Outport  Port=7
  SetNtcStsAndSnpshtData8 : Outport  Port=8

== system Ford_T3T6_ArchCnctnDigrm/Support Functions/ES101AProxy9_DiagcMgrProxy9 ==
  ClrDiagcFlgProxy : Inport
  DiagcMgrIninCore : Inport  Port=2
  GetNtcActvCore : Inport  Port=3
  GetNtcQlfrStsCore : Inport  Port=4
  GetNtcStsCore : Inport  Port=5
  SetNtcStsCore : Inport  Port=6
  GetDiagcDataAppl9 : Outport
  GetNtcActv9 : Outport  Port=2
  GetNtcDebCntrAppl9 : Outport  Port=3
  GetNtcInfoAppl9 : Outport  Port=4
  GetNtcQlfrSts9 : Outport  Port=5
  GetNtcSts9 : Outport  Port=6
  SetNtcSts9 : Outport  Port=7
  SetNtcStsAndSnpshtData9 : Outport  Port=8

== system Ford_T3T6_ArchCnctnDigrm/Support Functions/ES999A_ElecGlbPrm ==

== system Ford_T3T6_ArchCnctnDigrm/Support Functions/SF999A_SysGlbPrm ==

== system Ford_T3T6_ArchCnctnDigrm/System Diagnostic Action/ES101ACore_DiagcMgr ==
  BrdgVltg : Inport
  EcuTFild : Inport  Port=2
  HwTq : Inport  Port=3
  IgnCntr : Inport  Port=4
  MfgDiagcInhb : Inport  Port=5
  MfgEnaSt : Inport  Port=6
  MotTqCmdMrfScad : Inport  Port=7
  SwApplCrc : Inport  Port=8
  SysSt : Inport  Port=9
  Dem_ClearDTC : Inport  Port=10
  Dem_GetDTCOfEvent : Inport  Port=11
  Dem_SetEventStatus : Inport  Port=12
  DiagcMgrApplCrc_SetRamBlockStatus : Inport  Port=13
  DiagcMgrLtchCntrAry_SetRamBlockStatus : Inport  Port=14
  DiagcMgrNtcFltAry_SetRamBlockStatus : Inport  Port=15
  GetDiagcDataApplX : Inport  Port=16
  GetMcuDiagcSpplData : Inport  Port=17
  GetNtcDebCntrApplX : Inport  Port=18
  GetNtcInfoApplX : Inport  Port=19
  SnpshtDataAry_SetRamBlockStatus : Inport  Port=20
  ClrDiagcFlgProxy : Outport
  DiagcStsCtrldShtDwnFltPrsnt : Outport  Port=2
  DiagcStsNonRcvrlReqDiFltPrsnt : Outport  Port=3
  SysDiMotTqCmdSca : Outport  Port=4
  SysDiRampRate : Outport  Port=5
  SysStFltOutpReqDi : Outport  Port=6
  ClrAllDiagc : Outport  Port=7
  ClrLtchCntrData : Outport  Port=8
  ClrSnpshtData : Outport  Port=9
  CnvSnpshtData_f32 : Outport  Port=10
  CnvSnpshtData_logl : Outport  Port=11
  CnvSnpshtData_s08 : Outport  Port=12
  CnvSnpshtData_s16 : Outport  Port=13
  CnvSnpshtData_s32 : Outport  Port=14
  CnvSnpshtData_u08 : Outport  Port=15
  CnvSnpshtData_u16 : Outport  Port=16
  DiagcMgrIninCore : Outport  Port=17
  DiagcMgrPwrDwn : Outport  Port=18
  GetNtcActvCore : Outport  Port=19
  GetNtcQlfrStsCore : Outport  Port=20
  GetNtcStsCore : Outport  Port=21
  ReadLtchCntrData : Outport  Port=22
  ReadNtcFltAry : Outport  Port=23
  ReadNtcInfoAndDebCntr : Outport  Port=24
  ReadSnpshtData : Outport  Port=25
  RestoreDiagcMgrLtchCntrAryDft : Outport  Port=26
  RestoreNtcFltAryDft : Outport  Port=27
  RestoreSnpshtAryDft : Outport  Port=28
  SetNtcStsCore : Outport  Port=29
  UpdDtcEnaCdn : Outport  Port=30

== system Ford_T3T6_ArchCnctnDigrm/System Diagnostic Action/SF005A_StOutpCtrl ==
  DiagcStsCtrldShtDwnFltPrsnt : Inport
  LoaRateLim : Inport  Port=2
  LoaSca : Inport  Port=3
  MotTqTranlDampgCmpl : Inport  Port=4
  SysDiMotTqCmdSca : Inport  Port=5
  SysDiRampRate : Inport  Port=6
  SysMotTqCmdRampRateDi : Inport  Port=7
  SysOperMotTqCmdSca : Inport  Port=8
  SysOperRampRate : Inport  Port=9
  SysStFltOutpReqDi : Inport  Port=10
  VehStrtStopMotTqCmdSca : Inport  Port=11
  VehStrtStopRampRate : Inport  Port=12
  SysMotTqCmdSca : Outport
  SysStReqDi : Outport  Port=2

== system Ford_T3T6_ArchCnctnDigrm/System Wellness/CM111A_VrfyCritReg ==
  ClrErrInjReg : Inport
  MCalWrVrfyRegFltInfoStorg_GetErrorStatus : Inport  Port=2
  MCalWrVrfyRegFltInfoStorg_SetRamBlockStatus : Inport  Port=3
  ReadErrInjReg : Inport  Port=4
  SetNtcSts : Inport  Port=5
  InjVrfyCritRegErr : Outport
  MCalReadVrfyFailFltInfo : Outport  Port=2

== system Ford_T3T6_ArchCnctnDigrm/System Wellness/SF058B_SysOutpPrsntCpby ==
  BrdgVltg : Inport
  ImcSysSt : Inport  Port=2
  ImcSysStVld : Inport  Port=3
  MotBackEmfConEstimd : Inport  Port=4
  MotVelCrf : Inport  Port=5
  SysFricEstimd : Inport  Port=6
  SysSt : Inport  Port=7
  ThermMotTqLimCdnd : Inport  Port=8
  VehSpd : Inport  Port=9
  GetSigImcData_f32 : Inport  Port=10
  GetSigImcData_logl : Inport  Port=11
  EcuStsFlg : Outport
  FricFlg : Outport  Port=2
  MaxHwVel : Outport  Port=3
  MotKneePtTq : Outport  Port=4
  MotKneePtVel : Outport  Port=5
  MotTqAvl : Outport  Port=6
  MotZeroPtVel : Outport  Port=7
  ThermFlg : Outport  Port=8
  ThermFlgCombd : Outport  Port=9
  VltgFlg : Outport  Port=10
  VltgFlgCombd : Outport  Port=11

== system Ford_T3T6_ArchCnctnDigrm/Vector Components Base Software/AR001ADio_Dio ==

== system Ford_T3T6_ArchCnctnDigrm/Vector Components Base Software/AR001AEcuM_EcuM ==

== system Ford_T3T6_ArchCnctnDigrm/Vector Components Base Software/AR001AFls_Fls ==

== system Ford_T3T6_ArchCnctnDigrm/Vector Components Base Software/AR001APort_Port ==

== system Ford_T3T6_ArchCnctnDigrm/Vector Components Base Software/AR001ASpi_Spi ==
  Spi_AsyncTransmit : Outport
  Spi_GetSequenceResult : Outport  Port=2
  Spi_ReadIB : Outport  Port=3
  Spi_WriteIB : Outport  Port=4

== system Ford_T3T6_ArchCnctnDigrm/Vector Components Base Software/CAN ==

== system Ford_T3T6_ArchCnctnDigrm/Vector Components Base Software/COM ==
  AR001ACom_Com : Subsystem  Tag=0.0.X  Description=The AUTOSAR COM module is derived from OSEK/ VDX Communication Version 3.0.3. The AUTOSAR COM module provides signal gateway functionality. Main Features: - Provision of signal oriented data interface for the RTE, - Packing of AUTOSAR signals to I-PDUs to be transmitted, - Unpacking of received I-PDUs and provision of received signals to RTE, - Routing of signals from received I-PDUs into I-PDUs to become transmitted, - Routing of signal groups from received I-PDUs into I-PDUs to become transmitted, - Communication transmission control (start/ stop of I-PDU groups), - Replications of send requests, - Guarantee of minimum distances between transmit I-PDUs, - Monitoring of receive signals (signals timeout), - Filter mechanisms for incoming signals, - Different notification mechanisms, - Provision of init values and update indications, - Byte order conversion, - Sign extension, - Support of two different transmission modes per I-PDU, - Signal based gateway, - Support of large and dynamic length data types, - Support of I-PDU counters and I-PDU replication
      settings: AttributesFormatString=Version: %<Tag>
  AR001AIPduM_IPduM : Subsystem  Tag=0.0.X  Description=PDU multiplexing means using the same PCI (Protocol Control Information) of a PDU (Protocol Data Unit) with more than one unique layout of its SDU (Service Data Unit). A selector field is a piece of the SDU of the multiplexed PDU. It is used to distinguish the contents of the multiplexed PDUs from each other. Multiplexing of PDUs is currently known from CAN, but is not restricted to this communication system. On sender-side, the I-PDU Multiplexer module is responsible to combine appropriate I-PDUs from COM to new, multiplexed I-PDUs and send them back to the PDURouter. On receiver-side, it is responsible to interpret the content of multiplexed I-PDUs and provide COM with its appropriate separated I-PDUs taking into account the value of the selector field.
      settings: AttributesFormatString=Version: %<Tag>
  AR001APduR_PduR : Subsystem  Tag=0.0.X  Description=The PDU Router module provides services for routing of I-PDUs (Interaction Layer Protocol Data Units) using the following module types: Communication interface modules (e.g. Com, LinIf, CanIf, CanNm, FrIf and FrNm), Transport Protocol modules (e.g. J1939, LinTp [part of LinIf], CanTp, FrTp). The routing of I-PDUs are made statically by the I-PDU identifier, no I-PDUs are routed dynamically in run-time or dependent on contents. The location of the modules can be upper module (e.g. DCM, COM, IpduM) or a lower module (CanIf, FrIf, LinTp, IpduM, CanNm, FrNm). Note that the IpduM is listed as upper and lower module because it has two different roles (upper: Communication between COM module and IpduM module, lower: communication between IpduM module and communication interface module)
      settings: AttributesFormatString=Version: %<Tag>

== system Ford_T3T6_ArchCnctnDigrm/Vector Components Base Software/DIAG ==
  AR001ADcm_Dcm : Subsystem  Tag=0.0.X  Description=The DCM module provides a common API for diagnostic services. The functionality of the DCM module is used by external diagnostic tools during the development, manufacturing or service. The DCM module ensures diagnostic data flow and manages the diagnostic states, especially diagnostic sessions and security states. Furthermore, the DCM module checks if the diagnostic service request is supported and if the service may be executed in the current session according to the diagnostic states.
      settings: AttributesFormatString=Version: %<Tag>
  AR001ADem_Dem : Subsystem  Tag=0.0.X  Description=The service component Diagnostic Event Manager (Dem) is responsible for processing and storing diagnostic events (errors) and associated data. Further, the Dem provides fault information to the Dcm (e.g. read all stored DTCs from the event memory). The Dem offers interfaces to the application layer and to other BSW modules.
      settings: AttributesFormatString=Version: %<Tag>
  tag scope: Dem_ClearDTC=global, Dem_GetDTCOfEvent=global, Dem_GetEventStatus=global, Dem_GetIndicatorStatus=global, Dem_ReportErrorStatus=global, Dem_SetEventStatus=global
  wires:
  AR001ADem_Dem/1(Dem_ClearDTC) -> [Dem_ClearDTC]
  AR001ADem_Dem/2(Dem_GetDTCOfEvent) -> [Dem_GetDTCOfEvent]
  AR001ADem_Dem/3(Dem_GetEventStatus) -> [Dem_GetEventStatus]
  AR001ADem_Dem/4(Dem_GetIndicatorStatus) -> [Dem_GetIndicatorStatus]
  AR001ADem_Dem/5(Dem_ReportErrorStatus) -> [Dem_ReportErrorStatus]
  AR001ADem_Dem/6(Dem_SetEventStatus) -> [Dem_SetEventStatus]

== system Ford_T3T6_ArchCnctnDigrm/Vector Components Base Software/IO ==
  AR001A_IoHwAb : Subsystem  Tag=0.0.X  Description=The IO Hardware Abstraction module abstracts from the signal path of the ECU hardware (Layout, Microcontroller Pins, Microcontroller external devices like IO ASIC). It provides a signal based interface to the upper software layer. It performs static abstraction and inversion (if needed) of values according to their physical representation at the inputs/outputs of the ECU hardware (compensation of static influences caused within the path between ECU IO and Microcontroller pin, e.g. voltage divider, hardware inversion).
      settings: AttributesFormatString=Version: %<Tag>
  tag scope: IoHwAb_GetGpioEcuIdnPin1=global, IoHwAb_GetGpioEcuIdnPin2=global, IoHwAb_GetGpioMcuEna=global, IoHwAb_GetGpioMotDrvr0Diag=global, IoHwAb_GetGpioPwrOutpEnaFb=global, IoHwAb_SetFctGpioPhaALowrCmd=global, IoHwAb_SetFctGpioPhaAUpprCmd=global, IoHwAb_SetFctGpioPhaBLowrCmd=global, IoHwAb_SetFctGpioPhaBUpprCmd=global, IoHwAb_SetFctGpioPhaCLowrCmd=global, IoHwAb_SetFctGpioPhaCUpprCmd=global, IoHwAb_SetFctPrphlHwAg1=global, IoHwAb_SetFctPrphlHwTq1=global, IoHwAb_SetFctPrphlHwTq2=global, IoHwAb_SetFctPrphlPhaALowrCmd=global, IoHwAb_SetFctPrphlPhaAUpprCmd=global, IoHwAb_SetFctPrphlPhaBLowrCmd=global, IoHwAb_SetFctPrphlPhaBUpprCmd=global, IoHwAb_SetFctPrphlPhaCLowrCmd=global, IoHwAb_SetFctPrphlPhaCUpprCmd=global, IoHwAb_SetGpioGateDrv0Rst=global, IoHwAb_SetGpioPhaALowrCmd=global, IoHwAb_SetGpioPhaAUpprCmd=global, IoHwAb_SetGpioPhaBLowrCmd=global, IoHwAb_SetGpioPhaBUpprCmd=global, IoHwAb_SetGpioPhaCLowrCmd=global, IoHwAb_SetGpioPhaCUpprCmd=global, IoHwAb_SetGpioPwrTurnOffCtrl=global, IoHwAb_SetGpioSysFlt2A=global, IoHwAb_SetGpioTmplMonrWdg=global
  wires:
  AR001A_IoHwAb/1(IoHwAb_GetGpioEcuIdnPin1) -> [IoHwAb_GetGpioEcuIdnPin1]
  AR001A_IoHwAb/2(IoHwAb_GetGpioEcuIdnPin2) -> [IoHwAb_GetGpioEcuIdnPin2]
  AR001A_IoHwAb/3(IoHwAb_GetGpioMcuEna) -> [IoHwAb_GetGpioMcuEna]
  AR001A_IoHwAb/4(IoHwAb_GetGpioMotDrvr0Diag) -> [IoHwAb_GetGpioMotDrvr0Diag]
  AR001A_IoHwAb/5(IoHwAb_GetGpioPwrOutpEnaFb) -> [IoHwAb_GetGpioPwrOutpEnaFb]
  AR001A_IoHwAb/6(IoHwAb_SetFctGpioPhaALowrCmd) -> [IoHwAb_SetFctGpioPhaALowrCmd]
  AR001A_IoHwAb/7(IoHwAb_SetFctGpioPhaAUpprCmd) -> [IoHwAb_SetFctGpioPhaAUpprCmd]
  AR001A_IoHwAb/8(IoHwAb_SetFctGpioPhaBLowrCmd) -> [IoHwAb_SetFctGpioPhaBLowrCmd]
  AR001A_IoHwAb/9(IoHwAb_SetFctGpioPhaBUpprCmd) -> [IoHwAb_SetFctGpioPhaBUpprCmd]
  AR001A_IoHwAb/10(IoHwAb_SetFctGpioPhaCLowrCmd) -> [IoHwAb_SetFctGpioPhaCLowrCmd]
  AR001A_IoHwAb/11(IoHwAb_SetFctGpioPhaCUpprCmd) -> [IoHwAb_SetFctGpioPhaCUpprCmd]
  AR001A_IoHwAb/12(IoHwAb_SetFctPrphlHwAg1) -> [IoHwAb_SetFctPrphlHwAg1]
  AR001A_IoHwAb/13(IoHwAb_SetFctPrphlHwTq1) -> [IoHwAb_SetFctPrphlHwTq1]
  AR001A_IoHwAb/14(IoHwAb_SetFctPrphlHwTq2) -> [IoHwAb_SetFctPrphlHwTq2]
  AR001A_IoHwAb/15(IoHwAb_SetFctPrphlPhaALowrCmd) -> [IoHwAb_SetFctPrphlPhaALowrCmd]
  AR001A_IoHwAb/16(IoHwAb_SetFctPrphlPhaAUpprCmd) -> [IoHwAb_SetFctPrphlPhaAUpprCmd]
  AR001A_IoHwAb/17(IoHwAb_SetFctPrphlPhaBLowrCmd) -> [IoHwAb_SetFctPrphlPhaBLowrCmd]
  AR001A_IoHwAb/18(IoHwAb_SetFctPrphlPhaBUpprCmd) -> [IoHwAb_SetFctPrphlPhaBUpprCmd]
  AR001A_IoHwAb/19(IoHwAb_SetFctPrphlPhaCLowrCmd) -> [IoHwAb_SetFctPrphlPhaCLowrCmd]
  AR001A_IoHwAb/20(IoHwAb_SetFctPrphlPhaCUpprCmd) -> [IoHwAb_SetFctPrphlPhaCUpprCmd]
  AR001A_IoHwAb/21(IoHwAb_SetGpioGateDrv0Rst) -> [IoHwAb_SetGpioGateDrv0Rst]
  AR001A_IoHwAb/22(IoHwAb_SetGpioPhaALowrCmd) -> [IoHwAb_SetGpioPhaALowrCmd]
  AR001A_IoHwAb/23(IoHwAb_SetGpioPhaAUpprCmd) -> [IoHwAb_SetGpioPhaAUpprCmd]
  AR001A_IoHwAb/24(IoHwAb_SetGpioPhaBLowrCmd) -> [IoHwAb_SetGpioPhaBLowrCmd]
  AR001A_IoHwAb/25(IoHwAb_SetGpioPhaBUpprCmd) -> [IoHwAb_SetGpioPhaBUpprCmd]
  AR001A_IoHwAb/26(IoHwAb_SetGpioPhaCLowrCmd) -> [IoHwAb_SetGpioPhaCLowrCmd]
  AR001A_IoHwAb/27(IoHwAb_SetGpioPhaCUpprCmd) -> [IoHwAb_SetGpioPhaCUpprCmd]
  AR001A_IoHwAb/28(IoHwAb_SetGpioPwrTurnOffCtrl) -> [IoHwAb_SetGpioPwrTurnOffCtrl]
  AR001A_IoHwAb/29(IoHwAb_SetGpioSysFlt2A) -> [IoHwAb_SetGpioSysFlt2A]
  AR001A_IoHwAb/30(IoHwAb_SetGpioTmplMonrWdg) -> [IoHwAb_SetGpioTmplMonrWdg]

== system Ford_T3T6_ArchCnctnDigrm/Vector Components Base Software/MCAL ==
  AR001AMcu_Mcu : Subsystem  Tag=0.0.X  Description=The MCU driver provides services for basic microcontroller initialization, power down functionality, reset and microcontroller specific functions required by other MCAL software modules. The initialization services allow a flexible and application related MCU initialization in addition to the start-up code (see figure below). The start-up code is very MCU specific. The provided start-up code description in this document is for guidance and implies functionality which has to be taken into account before standardized MCU initialization is able to start.
      settings: AttributesFormatString=Version: %<Tag>
  AR001AWdg_Wdg : Subsystem  Tag=0.0.X  Description=This module provides services for initialization, changing the operation mode and setting the trigger condition (timeout).
      settings: AttributesFormatString=Version: %<Tag>
  tag scope: Mcu_PerformReset=global
  wires:
  AR001AMcu_Mcu/1(Mcu_PerformReset) -> [Mcu_PerformReset]

== system Ford_T3T6_ArchCnctnDigrm/Vector Components Base Software/MEM ==
  AR001AFee_Fee : Subsystem  Tag=0.0.X  Description=The Flash EEPROM Emulation (FEE) shall abstract from the device specific addressing scheme and segmentation and provide the upper layers with a virtual addressing scheme and segmentation as well as a ï¿½virtuallyï¿½ unlimited number of erase cycles.
      settings: AttributesFormatString=Version: %<Tag>
  AR001AMemIf_MemIf : Subsystem  Tag=0.0.X  Description=This module allows the NVRAM manager to access several memory abstraction modules (FEE or EA modules). The Memory Abstraction Interface (MemIf) shall abstract from the number of underlying FEE or EA modules and provide upper layers with a virtual segmentation on a uniform linear address space.
      settings: AttributesFormatString=Version: %<Tag>
  AR001ANvM_NvM : Subsystem  Tag=0.0.X  Description=The NvM module shall provide services to ensure the data storage and maintenance of NV (non volatile) data according to their individual requirements in an automotive environment. The NvM module shall be able to administrate the NV data of an EEPROM and/or a FLASH EEPROM emulation device. The NvM module shall provide the required synchronous/asynchronous services for the management and the maintenance of NV data (init/read/write/control).
      settings: AttributesFormatString=Version: %<Tag>
  tag scope: NvM_CancelWriteAll=global, NvM_GetErrorStatus=global, NvM_ReadAll=global, NvM_ReadBlock=global, NvM_SetRamBlockStatus=global, NvM_WriteAll=global, NvM_WriteBlock=global
  wires:
  AR001ANvM_NvM/1(NvM_CancelWriteAll) -> [NvM_CancelWriteAll]
  AR001ANvM_NvM/2(NvM_GetErrorStatus) -> [NvM_GetErrorStatus]
  AR001ANvM_NvM/3(NvM_ReadAll) -> [NvM_ReadAll]
  AR001ANvM_NvM/4(NvM_ReadBlock) -> [NvM_ReadBlock]
  AR001ANvM_NvM/5(NvM_SetRamBlockStatus) -> [NvM_SetRamBlockStatus]
  AR001ANvM_NvM/6(NvM_WriteAll) -> [NvM_WriteAll]
  AR001ANvM_NvM/7(NvM_WriteBlock) -> [NvM_WriteBlock]

== system Ford_T3T6_ArchCnctnDigrm/Vector Components Base Software/OS ==
